simulink model "gotowe"  (Simulink 7.5)
settings: Solver=ode45  StartTime=0.0  StopTime=T  RelTol=1e-3
undefined symbols (not defined in the file): b, c, Kr, ogr, Td, Tdf, Ti, Tp, Tt, yref
settings Model: Creator=sieklo  LastModifiedBy=Konrad

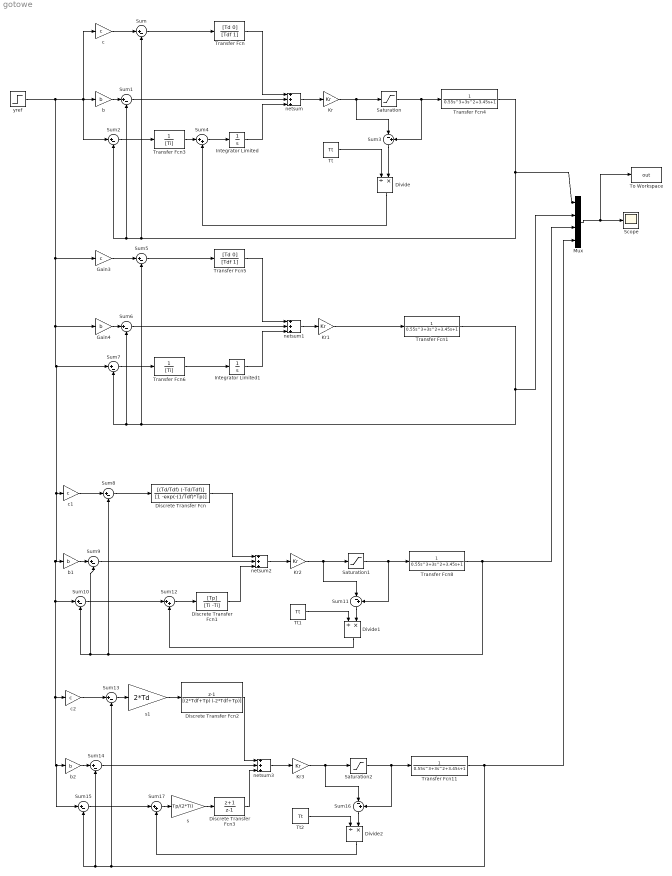
== system gotowe ==
  Discrete Transfer Fcn2 : DiscreteTransferFcn  Numerator=[1 -1]  Denominator=[(2*Tdf+Tp) (-2*Tdf+Tp)]  SampleTime=Tp
  Discrete Transfer Fcn3 : DiscreteTransferFcn  Numerator=[1 1]  Denominator=[1 -1]  SampleTime=Tp
  Discrete Transfer Fcn : DiscreteTransferFcn  Numerator=[(Td/Tdf) (-Td/Tdf)]  Denominator=[1 -exp(-(1/Tdf)*Tp)]  SampleTime=Tp
  Discrete Transfer Fcn1 : DiscreteTransferFcn  Numerator=[Tp]  Denominator=[Ti -Ti]  SampleTime=Tp
  Divide : Product  Inputs=/*
  Divide1 : Product  Inputs=/*
  Divide2 : Product  Inputs=/*
  Gain3 : Gain  Gain=c
  Gain4 : Gain  Gain=b
  Integrator Limited : Integrator  LimitOutput=on  UpperSaturationLimit=1  LowerSaturationLimit=-1
  Integrator Limited1 : Integrator  LimitOutput=on  UpperSaturationLimit=1  LowerSaturationLimit=-1
  Kr{,1..3} (4 alike) : Gain  Gain=Kr
  Mux : Mux
  Saturation : Saturate  UpperLimit=ogr  LowerLimit=-ogr
  Saturation1 : Saturate  UpperLimit=ogr  LowerLimit=-ogr
  Saturation2 : Saturate  UpperLimit=ogr  LowerLimit=-ogr
  Scope : Scope
  Sum{,1..2,5..10,13..15} (12 alike) : Sum  Inputs=|+-
  Sum11 : Sum  Inputs=|-+
  Sum12 : Sum  Inputs=|++
  Sum16 : Sum  Inputs=|-+
  Sum17 : Sum  Inputs=|++
  Sum3 : Sum  Inputs=|-+
  Sum4 : Sum  Inputs=|++
  To Workspace : ToWorkspace  VariableName=out  SampleTime=-1  SaveFormat=Structure
  Transfer Fcn : TransferFcn  Numerator=[Td 0]  Denominator=[Tdf 1]
  Transfer Fcn{1,4,8,11} (4 alike) : TransferFcn  Denominator=[0.55 3 3.45 1]
  Transfer Fcn3 : TransferFcn  Denominator=[Ti]
  Transfer Fcn5 : TransferFcn  Numerator=[Td 0]  Denominator=[Tdf 1]
  Transfer Fcn6 : TransferFcn  Denominator=[Ti]
  Tt : Constant  Value=Tt
  Tt1 : Constant  Value=Tt
  Tt2 : Constant  Value=Tt
  b : Gain  Gain=b
  b1 : Gain  Gain=b
  b2 : Gain  Gain=b
  c : Gain  Gain=c
  c1 : Gain  Gain=c
  c2 : Gain  Gain=c
  netsum{,1..3} (4 alike) : Sum  Inputs=3  SaturateOnIntegerOverflow=on  InputSameDT=on  OutDataTypeStr=Inherit: Same as first input
  s : Gain  Gain=Tp/(2*Ti)
  s1 : Gain  Gain=2*Td
  yref : Step  After=yref  SampleTime=0
  wires:
  Saturation/1 -> Transfer Fcn4/1, Sum3/2
  Sum/1 -> Transfer Fcn/1
  c/1 -> Sum/1
  b/1 -> Sum1/1
  Transfer Fcn/1 -> netsum/1
  Sum1/1 -> netsum/2
  netsum/1 -> Kr/1
  Kr/1 -> Saturation/1, Sum3/1
  yref/1 -> c/1, Sum2/1, b/1, Gain3/1, Gain4/1, Sum15/1, b2/1, c2/1, Sum10/1, b1/1, c1/1, Sum7/1
  Transfer Fcn4/1 -> Sum2/2, Sum1/2, Sum/2, Mux/1
  Integrator Limited/1 -> netsum/3
  Sum2/1 -> Transfer Fcn3/1
  Transfer Fcn3/1 -> Sum4/1
  Sum4/1 -> Integrator Limited/1
  Sum3/1 -> Divide/2
  Tt/1 -> Divide/1
  Divide/1 -> Sum4/2
  Mux/1 -> Scope/1, To Workspace/1
  Sum5/1 -> Transfer Fcn5/1
  Gain3/1 -> Sum5/1
  Gain4/1 -> Sum6/1
  Transfer Fcn5/1 -> netsum1/1
  Sum6/1 -> netsum1/2
  netsum1/1 -> Kr1/1
  Transfer Fcn1/1 -> Sum7/2, Sum6/2, Sum5/2, Mux/2
  Integrator Limited1/1 -> netsum1/3
  Sum7/1 -> Transfer Fcn6/1
  Transfer Fcn6/1 -> Integrator Limited1/1
  Kr1/1 -> Transfer Fcn1/1
  Saturation1/1 -> Transfer Fcn8/1, Sum11/2
  c1/1 -> Sum8/1
  b1/1 -> Sum9/1
  Sum9/1 -> netsum2/2
  netsum2/1 -> Kr2/1
  Kr2/1 -> Saturation1/1, Sum11/1
  Transfer Fcn8/1 -> Mux/3, Sum10/2, Sum9/2, Sum8/2
  Sum11/1 -> Divide1/2
  Tt1/1 -> Divide1/1
  Divide1/1 -> Sum12/2
  Saturation2/1 -> Transfer Fcn11/1, Sum16/2
  c2/1 -> Sum13/1
  b2/1 -> Sum14/1
  Sum14/1 -> netsum3/2
  netsum3/1 -> Kr3/1
  Kr3/1 -> Saturation2/1, Sum16/1
  Transfer Fcn11/1 -> Mux/4, Sum15/2, Sum14/2, Sum13/2
  Sum16/1 -> Divide2/2
  Tt2/1 -> Divide2/1
  Divide2/1 -> Sum17/2
  Discrete Transfer Fcn/1 -> netsum2/1
  Sum8/1 -> Discrete Transfer Fcn/1
  Sum13/1 -> s1/1
  s1/1 -> Discrete Transfer Fcn2/1
  Discrete Transfer Fcn2/1 -> netsum3/1
  Sum12/1 -> Discrete Transfer Fcn1/1
  Discrete Transfer Fcn1/1 -> netsum2/3
  Sum10/1 -> Sum12/1
  Sum15/1 -> Sum17/1
  Sum17/1 -> s/1
  s/1 -> Discrete Transfer Fcn3/1
  Discrete Transfer Fcn3/1 -> netsum3/3
